simulink model "dinamica2019"  (R2019b)
settings: Solver=VariableStepAuto  StartTime=0.0  StopTime=10.0  RelTol=1e-3
undefined symbols (not defined in the file or in its folder): g, l1, l2, m1, m2
settings Model: Creator=vfton  LastModifiedBy=vfton
settings DebuggingCC: UnconnectedInputMsg=none  UnconnectedOutputMsg=none  UnconnectedLineMsg=none  SFMachineParentedDataDiag=error

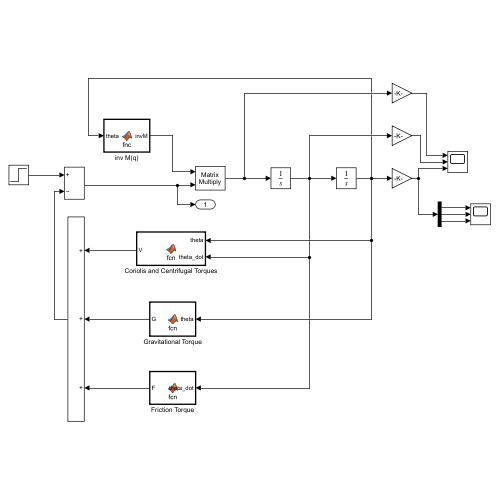
[thumbnail: Simulink's stored preview of the top-level diagram]
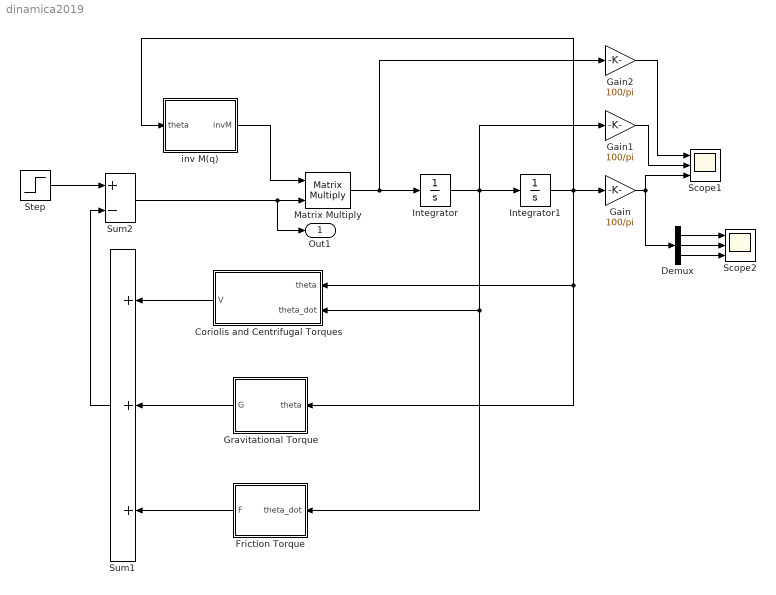
== system dinamica2019 ==
  "Coriolis and Centrifugal Torques " : MATLAB Function  TreatAsAtomicUnit=on
  Demux : Demux  Outputs=3
  Friction Torque : MATLAB Function  TreatAsAtomicUnit=on
  Gain : Gain  Gain=100/pi
  Gain1 : Gain  Gain=100/pi
  Gain2 : Gain  Gain=100/pi
  Gravitational Torque : MATLAB Function  TreatAsAtomicUnit=on
  Integrator : Integrator  InitialCondition=[0; 0; 0]
  Integrator1 : Integrator  InitialCondition=[0; 0; 0]
  Matrix Multiply : Product  Multiplication=Matrix(*)
  Scope1 : Scope  NumInputPorts=3
  Scope2 : Scope  NumInputPorts=3
  Step : Step  Before=[0; 0; 0]  After=[1; 0; 0]  SampleTime=0  VectorParams1D=off
  Sum1 : Sum  Inputs=+++
  Sum2 : Sum  Inputs=+-
  inv M(q) : MATLAB Function  TreatAsAtomicUnit=on
  Out1 : Outport
  wires:
  Step/1 -> Sum2/1
  Sum1/1 -> Sum2/2
  "Coriolis and Centrifugal Torques "/1(V) -> Sum1/1
  Gravitational Torque/1(G) -> Sum1/2
  Friction Torque/1(F) -> Sum1/3
  Sum2/1 -> Out1/1, Matrix Multiply/2
  Matrix Multiply/1 -> Gain2/1, Integrator/1
  Integrator/1 -> Friction Torque/1(theta_dot), "Coriolis and Centrifugal Torques "/2(theta_dot), Gain1/1, Integrator1/1
  Gain2/1 -> Scope1/1
  Gain/1 -> Demux/1, Scope1/3
  Gain1/1 -> Scope1/2
  Integrator1/1 -> inv M(q)/1(theta), Gravitational Torque/1(theta), "Coriolis and Centrifugal Torques "/1(theta), Gain/1
  Demux/1 -> Scope2/1
  Demux/3 -> Scope2/3
  Demux/2 -> Scope2/2
  inv M(q)/1(invM) -> Matrix Multiply/1

== matlab function dinamica2019/Gravitational Torque ==
  data: theta input size=[3,1]; G output size=[3,1]; m1 parameter; m2 parameter; l1 parameter; l2 parameter; g parameter
function G  = fcn(theta, m1, m2, l1, l2, g)
    G = zeros([3,1]);
    G(1) = m2*l2*g*cos(theta(1)+theta(2))+(m1+m2)*l1*g*cos(theta(1));
    G(2) = m2*l2*g*cos(theta(1)+theta(2));
    G(3) = 0;

== matlab function dinamica2019/Coriolis and Centrifugal Torques  ==
  data: theta input size=[3,1]; V output size=[3,1]; theta_dot input size=[3,1]; m2 parameter; l1 parameter; l2 parameter
function V  = fcn(theta,theta_dot,m2, l1, l2)
    V = zeros([3,1]);
    V(1) = -m2*l1*l2*sin(theta(2))*theta_dot(2)^2 - 2*m2*l1*l2*sin(theta(2))*theta_dot(1)*theta_dot(2);
    V(2) = m2*l1*l2*sin(theta(2))*theta_dot(1)^2;
    V(3) = 0;

== matlab function dinamica2019/Friction Torque ==
  data: theta_dot input size=[3,1]; F output size=[3,1]; v parameter
function F = fcn(theta_dot, v)
    F = zeros([3,1]);
    F(1) = v*theta_dot(1);
    F(2) = v*theta_dot(2);
    F(3) = 0;

== matlab function dinamica2019/inv M(q) ==
  data: theta input size=[3,1]; invM output size=[3,3]; m1 parameter; m2 parameter; l1 parameter; l2 parameter
function invM  = fnc(theta, m1, m2, l1, l2)
    M = zeros([3,3]);
    M(1,1) = m2*l2^2 + 2*m2*l1*l2*cos(theta(2))+(l1^2)*(m1+m2);
    M(1,2) = m2*l2^2 + m2*l1*l2*cos(theta(2));
    M(2,1) = m2*l2^2 + m2*l1*l2*cos(theta(2));
    M(2,2) = m2*l2^2;
    invM = inv(M);
